simulink model "ProdSystem_EOQAssumptionsAndCosts"  (R2015a)
settings: Solver=ode45  SolverMode=SingleTasking  StartTime=0  StopTime=10000000  RelTol=1e-3
libraries: simeventslib x8, simulink x1
settings Model: CovSFcnEnable=off  Creator=AnotherUser  LastModifiedBy=AnotherUser
settings OptimizationCC: BlockReduction=off  BooleanDataType=off
settings DebuggingCC: SaveWithParameterizedLinksMsg=none  UnderspecifiedInitializationDetection=Classic  MergeDetectMultiDrivingBlocksExec=none  SignalResolutionControl=TryResolveAllWithWarning
settings HardwareCC: TargetUnknown=on

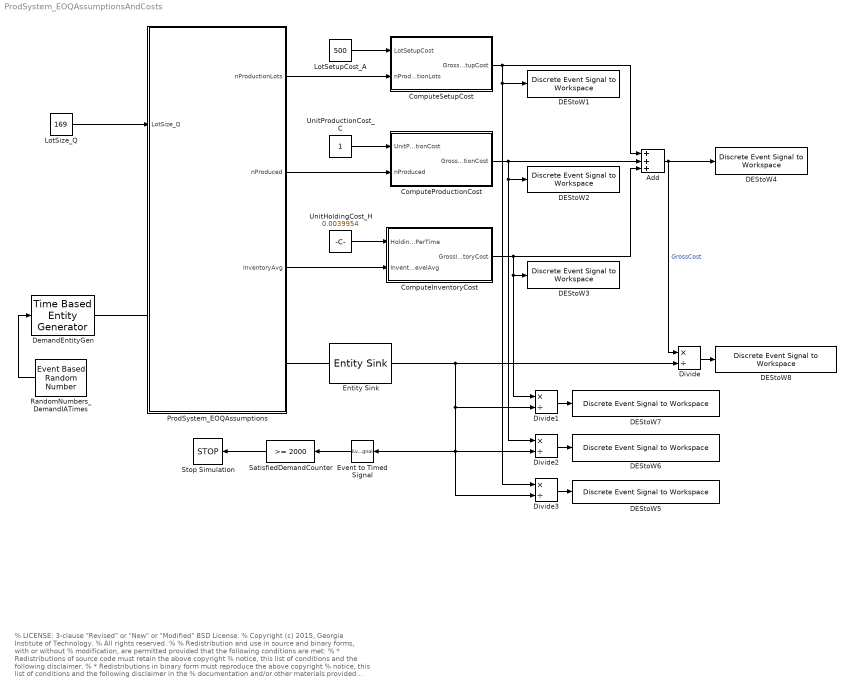
== system ProdSystem_EOQAssumptionsAndCosts ==
  note: % LICENSE: 3-clause "Revised" or "New" or "Modified" BSD License.
      | % Copyright (c) 2015, Georgia Institute of Technology.
      | % All rights reserved.
      | %
      | % Redistribution and use in source and binary forms, with or without
      | % modification, are permitted provided that the following conditions are met:
      | % * Redistributions of source code must retain the above copyright
      | % notice, this list of conditions and the following disclaimer.
      | % * Redistributions in binary form must reproduce the above copyright
      | % notice, this list of conditions and the following disclaimer in the
      | % documentation and/or other materials provided with the distribution.
      | % * Neither the name of the Georgia Institute of Technology nor the
      | % names of its contributors may be used to endorse or promote products
      | % derived from this software without specific prior written permission.
      | %
      | % THIS SOFTWARE IS PROVIDED BY THE COPYRIGHT HOLDERS AND CONTRIBUTORS "AS IS" AND
      | % ANY EXPRESS OR IMPLIED WARRANTIES, INCLUDING, BUT NOT LIMITED TO, THE IMPLIED
      | % WARRANTIES OF MERCHANTABILITY AND FITNESS FOR A PARTICULAR PURPOSE ARE
      | % DISCLAIMED. IN NO EVENT SHALL THE GEORGIA INSTITUTE OF TECHNOLOGY BE LIABLE FOR
      | % ANY DIRECT, INDIRECT, INCIDENTAL, SPECIAL, EXEMPLARY, OR CONSEQUENTIAL DAMAGES
      | % (INCLUDING, BUT NOT LIMITED TO, PROCUREMENT OF SUBSTITUTE GOODS OR SERVICES;
      | % LOSS OF USE, DATA, OR PROFITS; OR BUSINESS INTERRUPTION) HOWEVER CAUSED AND
      | % ON ANY THEORY OF LIABILITY, WHETHER IN CONTRACT, STRICT LIABILITY, OR TORT
      | % (INCLUDING NEGLIGENCE OR OTHERWISE) ARISING IN ANY WAY OUT OF THE USE OF THIS
      | % SOFTWARE, EVEN IF ADVISED OF THE POSSIBILITY OF SUCH DAMAGE.
  Add : Sum  Inputs=+++
  ComputeInventoryCost : Subsystem
  ComputeProductionCost : Subsystem
  ComputeSetupCost : Subsystem
  DEStoW1 : simeventslib/SimEvents Sinks/Discrete Event Signal to Workspace  VariableName=GrossSetupCost  SaveFormat=Structure With Time  isMonitorOnly=off  isRecordIC=off
  DEStoW2 : simeventslib/SimEvents Sinks/Discrete Event Signal to Workspace  VariableName=GrossProductionCost  SaveFormat=Structure With Time  isMonitorOnly=off  isRecordIC=off
  DEStoW3 : simeventslib/SimEvents Sinks/Discrete Event Signal to Workspace  VariableName=GrossInventoryCost  SaveFormat=Structure With Time  isMonitorOnly=off  isRecordIC=off
  DEStoW4 : simeventslib/SimEvents Sinks/Discrete Event Signal to Workspace  VariableName=GrossCost  SaveFormat=Structure With Time  isMonitorOnly=off  isRecordIC=off
  DEStoW5 : simeventslib/SimEvents Sinks/Discrete Event Signal to Workspace  VariableName=GrossSetupCost_PerSatDmd  SaveFormat=Structure With Time  isMonitorOnly=off  isRecordIC=off
  DEStoW6 : simeventslib/SimEvents Sinks/Discrete Event Signal to Workspace  VariableName=GrossProductionCost_PerSatDmd  SaveFormat=Structure With Time  isMonitorOnly=off  isRecordIC=off
  DEStoW7 : simeventslib/SimEvents Sinks/Discrete Event Signal to Workspace  VariableName=GrossInventoryCost_PerSatDmd  SaveFormat=Structure With Time  isMonitorOnly=off  isRecordIC=off
  DEStoW8 : simeventslib/SimEvents Sinks/Discrete Event Signal to Workspace  VariableName=GrossCost_PerSatDmd  SaveFormat=Structure With Time  isMonitorOnly=off  isRecordIC=off
  DemandEntityGen : TimeBasedEntityGenerator  GenerateEntitiesUpon=Intergeneration time from port t  GenerateEntityAtSimulationStart=off
  Divide{,1..3} (4 alike) : Product  Inputs=*/
  Entity Sink : EntitySink  StatNumberArrived=on
  Event to Timed Signal : EventToTimedSignal
  LotSetupCost_A : Constant  Value=500
  LotSize_Q : Constant  Value=169
  ProdSystem_EOQAssumptions : Subsystem
  RandomNumbers_DemandIATimes : EventBasedRandomNumber  Distribution=Gamma  meanExp=8.76  scaleGam=17.52  shapeGam=0.5  meanNorm=8.76  stdNorm=1.3053e-07  scaleLogn=2.1702  shapeLogn=1.4901e-08  Seed=13103
  SatisfiedDemandCounter : simulink/Logic and Bit Operations/Compare To Constant  relop=>=  const=2000  OutDataTypeStr=boolean
  Stop Simulation : Stop
  UnitHoldingCost_H : Constant  Value=0.0039954
  UnitProductionCost_C : Constant
  wires:
  LotSize_Q/1 -> ProdSystem_EOQAssumptions/1(LotSize_Q)
  ComputeProductionCost/1(GrossProductionCost) -> Divide2/1, DEStoW2/1, Add/2
  ComputeSetupCost/1(GrossSetupCost) -> Divide3/1, DEStoW1/1, Add/1
  ComputeInventoryCost/1(GrossInventoryCost) -> Add/3, DEStoW3/1, Divide1/1
  Add/1 -> Divide/1, DEStoW4/1  "GrossCost"
  Divide/1 -> DEStoW8/1
  RandomNumbers_DemandIATimes/1 -> DemandEntityGen/1
  Divide1/1 -> DEStoW7/1
  Divide2/1 -> DEStoW6/1
  Divide3/1 -> DEStoW5/1
  Entity Sink/1 -> Divide1/2, Event to Timed Signal/1, Divide3/2, Divide2/2, Divide/2
  Event to Timed Signal/1 -> SatisfiedDemandCounter/1
  SatisfiedDemandCounter/1 -> Stop Simulation/1
  ProdSystem_EOQAssumptions/1(nProductionLots) -> ComputeSetupCost/2(nProductionLots)
  LotSetupCost_A/1 -> ComputeSetupCost/1(LotSetupCost)
  ProdSystem_EOQAssumptions/2(nProduced) -> ComputeProductionCost/2(nProduced)
  UnitProductionCost_C/1 -> ComputeProductionCost/1(UnitProductionCost)
  ProdSystem_EOQAssumptions/3(InventoryAvg) -> ComputeInventoryCost/2(InventoryLevelAvg)
  UnitHoldingCost_H/1 -> ComputeInventoryCost/1(HoldingCost_PerUnitPerTime)
  connections:
  DemandEntityGen/RConn1 -- ProdSystem_EOQAssumptions/LConn1
  ProdSystem_EOQAssumptions/RConn1 -- Entity Sink/LConn1

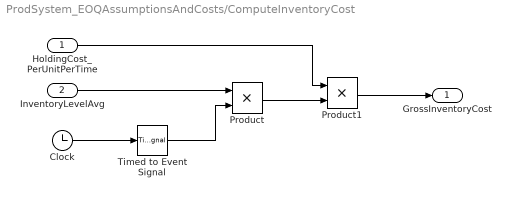
== system ProdSystem_EOQAssumptionsAndCosts/ComputeInventoryCost ==
  HoldingCost_PerUnitPerTime : Inport
  InventoryLevelAvg : Inport  Port=2
  Clock : Clock
  Product : Product
  Product1 : Product
  Timed to Event Signal : TimedToEventSignal
  GrossInventoryCost : Outport
  wires:
  Clock/1 -> Timed to Event Signal/1
  Timed to Event Signal/1 -> Product/2
  InventoryLevelAvg/1 -> Product/1
  Product/1 -> Product1/2
  HoldingCost_PerUnitPerTime/1 -> Product1/1
  Product1/1 -> GrossInventoryCost/1

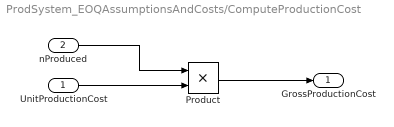
== system ProdSystem_EOQAssumptionsAndCosts/ComputeProductionCost ==
  UnitProductionCost : Inport
  nProduced : Inport  Port=2
  Product : Product
  GrossProductionCost : Outport
  wires:
  nProduced/1 -> Product/1
  UnitProductionCost/1 -> Product/2
  Product/1 -> GrossProductionCost/1

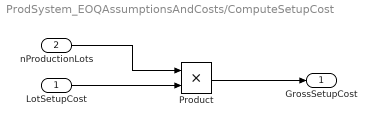
== system ProdSystem_EOQAssumptionsAndCosts/ComputeSetupCost ==
  LotSetupCost : Inport
  nProductionLots : Inport  Port=2
  Product : Product
  GrossSetupCost : Outport
  wires:
  nProductionLots/1 -> Product/1
  LotSetupCost/1 -> Product/2
  Product/1 -> GrossSetupCost/1

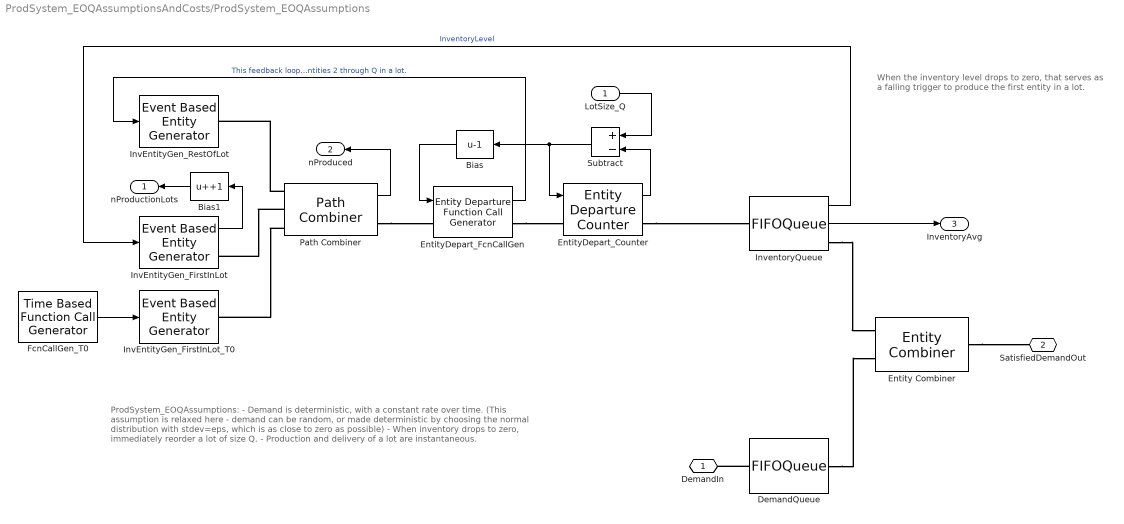
== system ProdSystem_EOQAssumptionsAndCosts/ProdSystem_EOQAssumptions ==
  note: When the inventory level drops to zero,
      | that serves as a falling trigger to produce
      | the first entity in a lot.
  note: ProdSystem_EOQAssumptions:
      |
      | - Demand is deterministic, with a constant rate over time.
      | (This assumption is relaxed here - demand can be random, or made deterministic by
      | choosing the normal distribution with stdev=eps, which is as close to zero as possible)
      |
      | - When inventory drops to zero, immediately reorder a lot of size Q.
      |
      | - Production and delivery of a lot are instantaneous.
  LotSize_Q : Inport
  Bias : Bias  Bias=-1
  Bias1 : Bias  Bias=+1
  DemandQueue : FIFOQueue  Capacity=Inf
  Entity Combiner : EntityCombiner  NumberInputPorts=2  AttributeAccessibility=off  TimerAccessibility=off
  EntityDepart_Counter : EntityDepartureCounter  NumberDepartedToSignal=on  NumberDepartedToAttribute=off  CounterResetTypeOption=Trigger from port tr  CounterResetEdgeOption=Falling
  EntityDepart_FcnCallGen : EntityDepartureFunctionCallGenerator  EnableE1Port=on
  FcnCallGen_T0 : TimeBasedFunctionCallGenerator  EventGenerationMode=Only at simulation start
  InvEntityGen_FirstInLot : EventBasedEntityGenerator  GenerateEntitiesUpon=Trigger from port tr  SignalEdgeType=Falling  StatNumberDeparted=on
  InvEntityGen_FirstInLot_T0 : EventBasedEntityGenerator  GenerateEntitiesUpon=Function call from port fcn
  InvEntityGen_RestOfLot : EventBasedEntityGenerator  GenerateEntitiesUpon=Function call from port fcn
  InventoryQueue : FIFOQueue  Capacity=Inf  StatNumberInBlock=on  StatAverageQueueLength=on
      settings: OutputPortMap=o1,o3
  Path Combiner : PathCombiner  StatNumberDeparted=on
  Subtract : Sum  Inputs=+-
  DemandIn : PMIOPort  Port=1  Side=Left
  SatisfiedDemandOut : PMIOPort  Port=2  Side=Right
  nProductionLots : Outport
  nProduced : Outport  Port=2
  InventoryAvg : Outport  Port=3
  wires:
  EntityDepart_FcnCallGen/1 -> InvEntityGen_RestOfLot/1  "This feedback loop produces entities 2 through Q in a lot."
  Subtract/1 -> EntityDepart_Counter/1, Bias/1
  InventoryQueue/1 -> InvEntityGen_FirstInLot/1  "InventoryLevel"
  FcnCallGen_T0/1 -> InvEntityGen_FirstInLot_T0/1
  Bias/1 -> EntityDepart_FcnCallGen/1
  EntityDepart_Counter/1 -> Subtract/2
  LotSize_Q/1 -> Subtract/1
  Path Combiner/1 -> nProduced/1
  Bias1/1 -> nProductionLots/1
  InvEntityGen_FirstInLot/1 -> Bias1/1
  InventoryQueue/2 -> InventoryAvg/1
  connections:
  Path Combiner/RConn1 -- EntityDepart_FcnCallGen/LConn1
  EntityDepart_Counter/RConn1 -- InventoryQueue/LConn1
  EntityDepart_FcnCallGen/RConn1 -- EntityDepart_Counter/LConn1
  DemandQueue/RConn1 -- Entity Combiner/LConn2
  Path Combiner/LConn3 -- InvEntityGen_FirstInLot_T0/RConn1
  Path Combiner/LConn2 -- InvEntityGen_FirstInLot/RConn1
  Path Combiner/LConn1 -- InvEntityGen_RestOfLot/RConn1
  InventoryQueue/RConn1 -- Entity Combiner/LConn1
  DemandQueue/LConn1 -- DemandIn/RConn1
  Entity Combiner/RConn1 -- SatisfiedDemandOut/RConn1
